simulink model "Atmosphere_Model"  (R2024b)
settings: Solver=VariableStepAuto  StartTime=0.0  StopTime=10.0  RelTol=1e-3
undefined symbols (not defined in the file or in its folder): m, s
libraries: aerolibasang x3, aerolibatmos2 x1, aerolibconvert2 x1
settings Model: Creator=lisav  LastModifiedBy=lisav

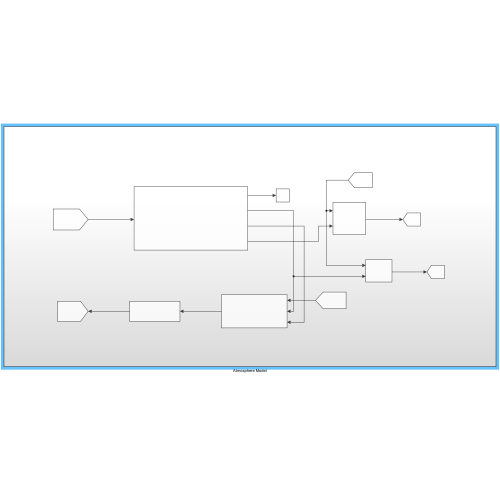
[thumbnail: Simulink's stored preview of the top-level diagram]
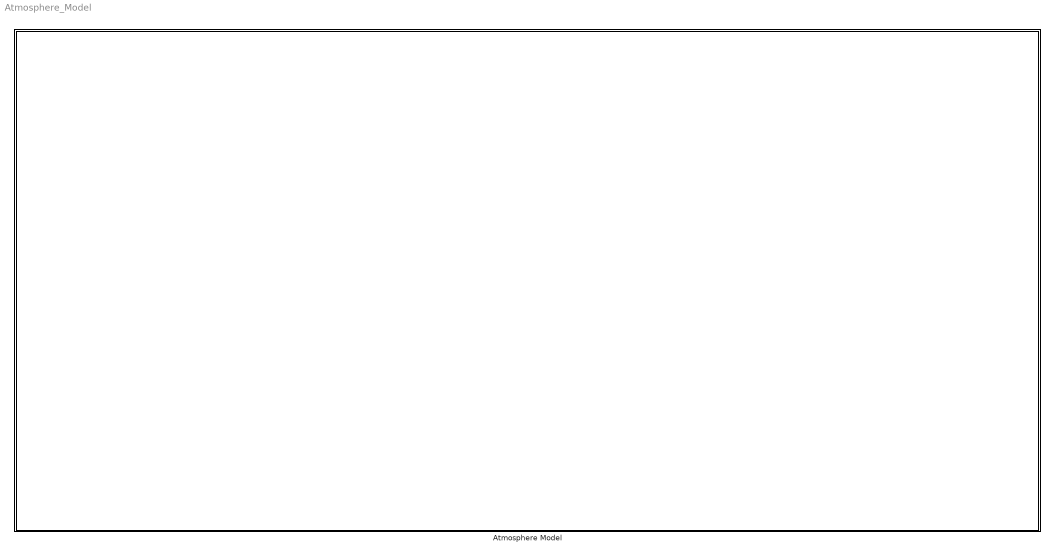
== system Atmosphere_Model ==
  Atmosphere Model : Subsystem

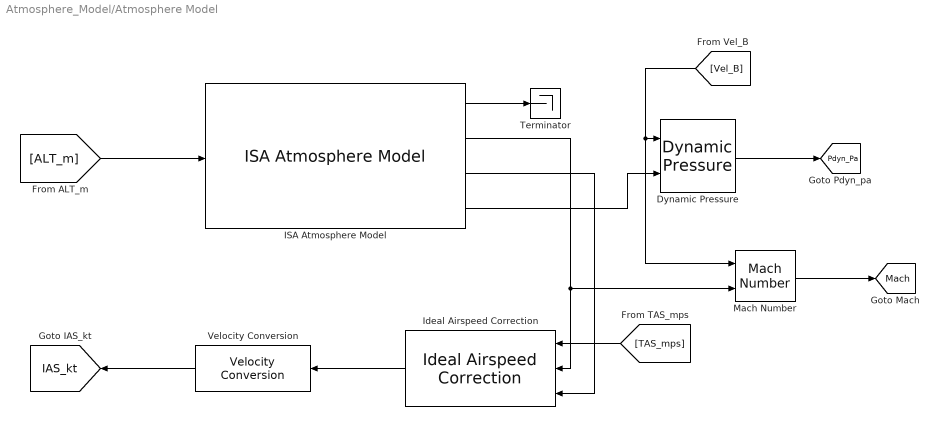
== system Atmosphere_Model/Atmosphere Model ==
  Dynamic Pressure : aerolibasang/Dynamic Pressure
  ISA Atmosphere Model : aerolibatmos2/ISA Atmosphere Model  useExtended=off  action=Warning  custom=off  viscosityOut=off  g=9.80665  gamma=1.4  R=287.0531  L=0.0065  h_trop=11000  h_strat=20000  rho0=1.225  P0=101325  T0=288.15  h0=0  S=110.4  Tref=273.15  muref=1.716e-5
  Ideal Airspeed Correction : aerolibasang/Ideal Airspeed Correction  units=Metric (MKS)  vel_in=TAS  vel_out_tas=EAS  vel_out_eas=TAS  vel_out_cas=TAS  method=Table Lookup  SubOnly=off  action=None
  Mach Number : aerolibasang/Mach Number
  Terminator : Terminator
  Velocity Conversion : aerolibconvert2/Velocity Conversion  IU=m/s  OU=kts
  tag scope: IAS_kt=global, Mach=global, Pdyn_Pa=global
  wires:
  Velocity Conversion/1 -> [IAS_kt]
  ISA Atmosphere Model/1 -> Terminator/1
  ISA Atmosphere Model/4 -> Dynamic Pressure/2
  [Vel_B] -> Mach Number/1, Dynamic Pressure/1
  [ALT_m] -> ISA Atmosphere Model/1
  Mach Number/1 -> [Mach]
  Dynamic Pressure/1 -> [Pdyn_Pa]
  ISA Atmosphere Model/3 -> Ideal Airspeed Correction/3
  [TAS_mps] -> Ideal Airspeed Correction/1
  ISA Atmosphere Model/2 -> Mach Number/2, Ideal Airspeed Correction/2
  Ideal Airspeed Correction/1 -> Velocity Conversion/1
